simulink model "version5"  (R2018b)
settings: Solver=FixedStepAuto  StartTime=0.0  StopTime=1  FixedStep=0.0005  RelTol=1e-3  EnableMultiTasking=on
model workspace (MAT data in the model file):
  APPS_1_X = [526 863 1200 1537 1837 2212 2310]
  APPS_2_X = [0 342 684 1026 1368 1710 1805]
  APPS_Y = [100 80 60 40 20 0 0]
  Motor_Temp = [0 25 50 75 85 100 115 125 150 175 200 225 250]
  duty_time = [0 1000 5000 6500 7500 9000 10000 10000 10000 10000 10000 10000 10000]
undefined symbols (not defined in the file): I_AN06_5V, I_AN08_5V, I_AN09_5V, I_HALL1, I_SW11_H, O_PWM1_LS0A7, O_PWM2_LS0A7, O_SW01_LS0A4
libraries: ec5744lib x55, simulink x28, canmsglib x12, fuzblock x2
(part 1 of 3)
settings Model: Creator=Hiro  LastModifiedBy=Hiro
settings SolverCC: AutoInsertRateTranBlk=on
settings DataIOCC: LimitDataPoints=on  SaveFormat=Array
settings OptimizationCC: DefaultParameterBehavior=Inlined  InlineInvariantSignals=on  EnhancedBackFolding=on  ExpressionFolding=off  PassReuseOutputArgsAs=Individual arguments  RollThreshold=65  StateBitsets=on  DataBitsets=on  ZeroExternalMemoryAtStartup=off  ZeroInternalMemoryAtStartup=off  EfficientFloat2IntCast=on  OptimizeBlockOrder=speed  DifferentSizesBufferReuse=on
settings DebuggingCC: SolverPrmCheckMsg=warning  InheritedTsInSrcMsg=none  ParameterTunabilityLossMsg=error  SFUnexpectedBacktrackingDiag=warning  SFNoUnconditionalDefaultTransitionDiag=warning  SFExecutionAtInitializationDiag=none
settings HardwareCC: ProdBitPerPointer=32  ProdBitPerSizeT=32  ProdBitPerPtrDiffT=32  ProdLargestAtomicInteger=Long  ProdLargestAtomicFloat=Double  ProdEndianess=BigEndian  ProdWordSize=32  ProdHWDeviceType=Freescale MPC5500
settings ModelReferenceCC: PropagateSignalLabelsOutOfModel=off
settings SFSimCC: SimUseLocalCustomCode=off  MATLABDynamicMemAlloc=off
settings RTWCC: SystemTargetFile=ec5744.tlc  MakeCommand=make_rtw optimized_fixed_point=1  GenerateMakefile=off  TemplateMakefile=ec5744_lcc.tmf  Description=Target for EC5744  GenerateReport=on  RTWUseLocalCustomCode=off  IncludeHyperlinkInReport=on  LaunchReport=on  GenerateTraceInfo=on  GenerateTraceReport=on  GenerateTraceReportSl=on  GenerateTraceReportSf=on  GenerateTraceReportEml=on
settings CodeAppCC: ForceParamTrailComments=on  IgnoreCustomStorageClasses=off  OperatorAnnotations=on  SimulinkDataObjDesc=on  SFDataObjDesc=on  InsertBlockDesc=on
settings STFCustomTargetCC: MultiwordLength=256  ModelReferenceCompliant=off  IncludeMdlTerminateFcn=off  CombineOutputUpdateFcns=on  SuppressErrorStatus=on  ERTCustomFileBanners=on  SupportContinuousTime=off  SupportNonInlinedSFcns=off  RemoveResetFunc=on  MATLABClassNameForMDSCustomization=Simulink.SoftwareTarget.ERTCustomization  SystemTargetFile=ec5744.tlc
settings ERTTargetCC: ModelReferenceCompliant=off  ParMdlRefBuildCompliant=off  CompOptLevelCompliant=off  ConcurrentExecutionCompliant=off  IncludeMdlTerminateFcn=off  SuppressErrorStatus=on  ModelStepFunctionPrototypeControlCompliant=off  CPPClassGenCompliant=off  UseToolchainInfoCompliant=off  GenerateASAP2=on  InlinedParameterPlacement=NonHierarchical  ERTSrcFileBannerTemplate=ec5744_code_template.cgt  ERTHdrFileBannerTemplate=ec5744_code_template.cgt  ERTDataSrcFileTemplate=ec5744_code_template.cgt  ERTDataHdrFileTemplate=ec5744_code_template.cgt  ERTCustomFileTemplate=ec5744_file_process.tlc
settings ConfigComp: CovMetricSettings=dw  CovHtmlReporting=on  CovSaveCumulativeToWorkspaceVar=on  CovSaveSingleToWorkspaceVar=on  CovExternalEMLEnable=off  CovSFcnEnable=off

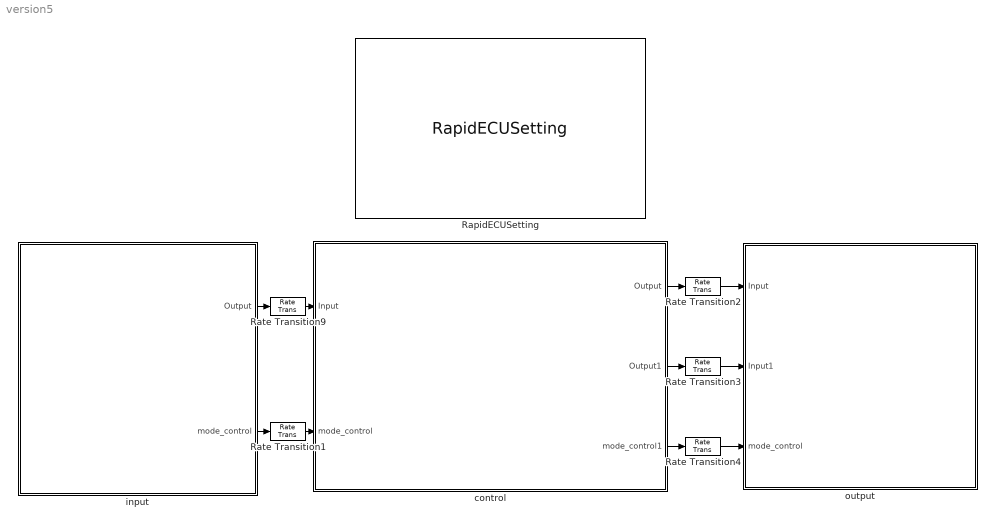
== system version5 ==
  RapidECUSetting : ec5744lib/RapidECU_U3/RapidECUSetting
      settings: SourceProductName=ECUCoder for MPC5744
  Rate Transition{1..4,9} (5 alike) : RateTransition  Integrity=off
  control : Subsystem
  input : Subsystem
  output : Subsystem
  wires:
  control/1(Output) -> Rate Transition2/1
  control/3(mode_control1) -> Rate Transition4/1
  control/2(Output1) -> Rate Transition3/1
  input/1(Output) -> Rate Transition9/1
  Rate Transition9/1 -> control/1(Input)
  input/2(mode_control) -> Rate Transition1/1
  Rate Transition1/1 -> control/2(mode_control)
  Rate Transition2/1 -> output/1(Input)
  Rate Transition3/1 -> output/2(Input1)
  Rate Transition4/1 -> output/3(mode_control)

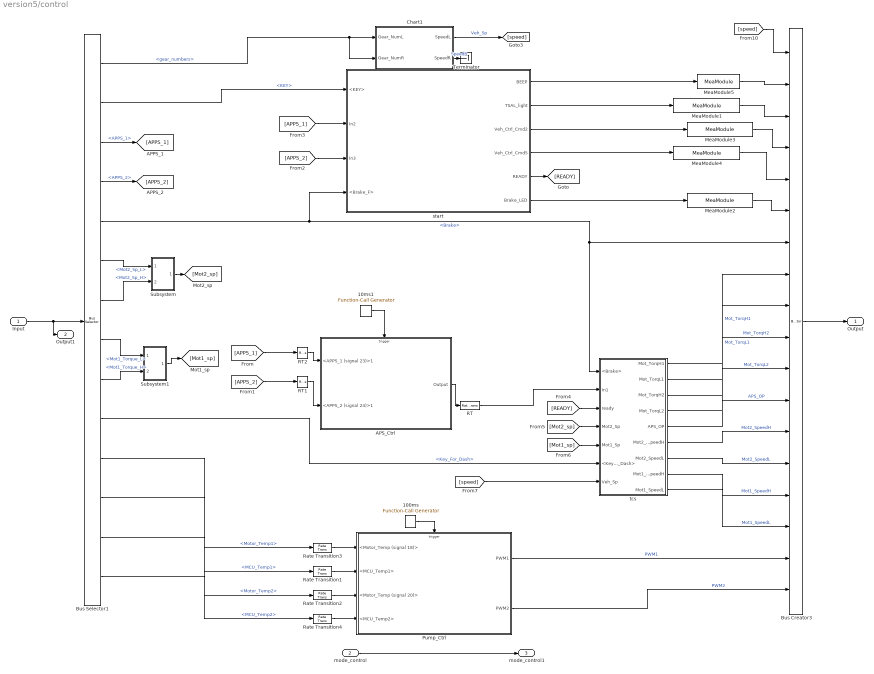
== system version5/control ==
  Input : Inport
  mode_control : Inport  Port=2
  100ms : simulink/Ports & Subsystems/Function-Call Generator  sample_time=0.1  numberOfIterations=1
  10ms1 : simulink/Ports & Subsystems/Function-Call Generator  sample_time=0.01  numberOfIterations=1
  APS_Ctrl : Subsystem
  Bus Creator3 : BusCreator  Inputs=18
  Bus Selector1 : BusSelector  OutputSignals=gear_numbers,KEY,APPS_1,APPS_2,Brake,Mot2_Sp_L,Mot2_Sp_H,Mot1_Torque_L,Mot1_Torque_H,Key_For_Dash,Motor_Temp1,MCU_Temp1,Motor_Temp2,MCU_Temp2
  Chart1 : Stateflow chart  TreatAsAtomicUnit=on
  MeaModule1 : ec5744lib/RapidECU_U3/07Calibration/MeaModule  signal=TSAL_LIGHT
      settings: SourceProductName=ECUCoder for MPC5744
  MeaModule2 : ec5744lib/RapidECU_U3/07Calibration/MeaModule  signal=Brake_LED
      settings: SourceProductName=ECUCoder for MPC5744
  MeaModule3 : ec5744lib/RapidECU_U3/07Calibration/MeaModule  signal=Veh_Ctrl_Cmd2
      settings: SourceProductName=ECUCoder for MPC5744
  MeaModule4 : ec5744lib/RapidECU_U3/07Calibration/MeaModule  signal=Veh_Ctrl_Cmd5
      settings: SourceProductName=ECUCoder for MPC5744
  MeaModule5 : ec5744lib/RapidECU_U3/07Calibration/MeaModule  signal=BEEP
      settings: SourceProductName=ECUCoder for MPC5744
  Pump_Ctrl : Subsystem
  RT : RateTransition  OutPortSampleTime=0.0005
  RT1 : RateTransition  OutPortSampleTime=0.01
  RT2 : RateTransition  OutPortSampleTime=0.01
  Rate Transition{1..4} (4 alike) : RateTransition  Integrity=off
  Subsystem : Subsystem
  Subsystem1 : Subsystem
  Terminator : Terminator
  start : Subsystem
  tcs : Subsystem
  Output : Outport
  Output1 : Outport  Port=2
  mode_control1 : Outport  Port=3
  wires:
  Pump_Ctrl/1(PWM1) -> Bus Creator3/17  "PWM1"
  Pump_Ctrl/2(PWM2) -> Bus Creator3/18  "PWM2"
  Input/1 -> Bus Selector1/1, Output1/1
  MeaModule1/1 -> Bus Creator3/3
  MeaModule2/1 -> Bus Creator3/6
  [APPS_1] -> RT2/1
  [APPS_2] -> RT1/1
  Bus Creator3/1 -> Output/1
  Bus Selector1/5 -> tcs/1(<Brake>), Bus Creator3/7, start/4(<Brake_F>)  "<Brake>"
  Bus Selector1/3 -> [APPS_1]  "<APPS_1>"
  Bus Selector1/4 -> [APPS_2]  "<APPS_2>"
  Bus Selector1/11 -> Rate Transition3/1  "<Motor_Temp1>"
  Bus Selector1/13 -> Rate Transition2/1  "<Motor_Temp2>"
  MeaModule3/1 -> Bus Creator3/4
  MeaModule4/1 -> Bus Creator3/5
  10ms1/1 -> APS_Ctrl/Trigger
  Bus Selector1/12 -> Rate Transition1/1  "<MCU_Temp1>"
  Bus Selector1/14 -> Rate Transition4/1  "<MCU_Temp2>"
  MeaModule5/1 -> Bus Creator3/2
  Bus Selector1/10 -> tcs/6(<Key_For_Dash>)  "<Key_For_Dash>"
  Bus Selector1/6 -> Subsystem/1(<Mot2_Sp_L>)  "<Mot2_Sp_L>"
  Bus Selector1/7 -> Subsystem/2(<Mot2_Sp_H>)  "<Mot2_Sp_H>"
  Bus Selector1/8 -> Subsystem1/1(<Mot1_Sp_L>)  "<Mot1_Torque_L>"
  Bus Selector1/9 -> Subsystem1/2(<Mot1_Sp_H>)  "<Mot1_Torque_H>"
  RT/1 -> tcs/2(In1)
  [READY] -> tcs/3(ready)
  [speed] -> tcs/7(Veh_Sp)
  tcs/1(Mot_TorqH1) -> Bus Creator3/8  "Mot_TorqH1"
  tcs/2(Mot_TorqL1) -> Bus Creator3/9  "Mot_TorqL1"
  tcs/5(APS_OP) -> Bus Creator3/12  "APS_OP"
  Subsystem/1(Mot2_Sp) -> [Mot2_sp]
  Subsystem1/1(Mot1_Sp) -> [Mot1_sp]
  [Mot2_sp] -> tcs/4(Mot2_Sp)
  [Mot1_sp] -> tcs/5(Mot1_Sp)
  mode_control/1 -> mode_control1/1
  tcs/6(Mot2_SpeedH) -> Bus Creator3/13  "Mot2_SpeedH"
  tcs/7(Mot2_SpeedL) -> Bus Creator3/14  "Mot2_SpeedL"
  tcs/8(Mot1_SpeedH) -> Bus Creator3/15  "Mot1_SpeedH"
  tcs/9(Mot1_SpeedL) -> Bus Creator3/16  "Mot1_SpeedL"
  100ms/1 -> Pump_Ctrl/Trigger
  Rate Transition3/1 -> Pump_Ctrl/1(<Motor_Temp (signal 18)>)
  Rate Transition1/1 -> Pump_Ctrl/2(<MCU_Temp1>)
  Rate Transition2/1 -> Pump_Ctrl/3(<Motor_Temp (signal 20)>)
  Rate Transition4/1 -> Pump_Ctrl/4(<MCU_Temp2>)
  Bus Selector1/2 -> start/1(<KEY>)  "<KEY>"
  [APPS_1] -> start/2(In2)
  [APPS_2] -> start/3(In3)
  start/1(BEEP) -> MeaModule5/1
  start/2(TSAL_light) -> MeaModule1/1
  start/3(Veh_Ctrl_Cmd2) -> MeaModule3/1
  start/4(Veh_Ctrl_Cmd5) -> MeaModule4/1
  start/5(READY) -> [READY]
  Chart1/1(SpeedL) -> [speed]  "Veh_Sp"
  [speed] -> Bus Creator3/1
  start/6(Brake_LED) -> MeaModule2/1
  tcs/3(Mot_TorqH2) -> Bus Creator3/10  "Mot_TorqH2"
  tcs/4(Mot_TorqL2) -> Bus Creator3/11  "Mot_TorqL2"
  APS_Ctrl/1(Output) -> RT/1
  RT1/1 -> APS_Ctrl/2(<APPS_2 (signal 24)>1)
  RT2/1 -> APS_Ctrl/1(<APPS_1 (signal 23)>1)
  Bus Selector1/1 -> Chart1/2(Gear_NumR), Chart1/1(Gear_NumL)  "<gear_numbers>"
  Chart1/2(SpeedR) -> Terminator/1  "SpeedR"

== system version5/input ==
  note: AnalogInput
  note: DASHtoVCU
  note: MCUtoVCU2
  note: BMStoVCU
  note: MCU to VCU1
  AnalogInput : Subsystem
  BMStoVCU : Subsystem
  Bus Creator : BusCreator  Inputs=27
  DASHtoVCU : Subsystem
  FrequencyRead1 : ec5744lib/RapidECU_U3/01BasicInput/FrequencyRead  channel=37:I_HALL1  sampletime=-1
      settings: SourceProductName=ECUCoder for MPC5744
  MCU to VCU : Subsystem
  MCUtoVCU : Subsystem
  SwitchInput : ec5744lib/RapidECU_U3/01BasicInput/SwitchInput  channel=44:I_SW11_H  sampletime=-1
      settings: SourceProductName=ECUCoder for MPC5744
  Output : Outport
  mode_control : Outport  Port=2
  wires:
  SwitchInput/1 -> Bus Creator/26  "KEY"
  Bus Creator/1 -> Output/1
  AnalogInput/1(Brake) -> Bus Creator/23
  AnalogInput/2(APPS_1) -> Bus Creator/24
  AnalogInput/3(APPS_2) -> Bus Creator/25
  MCU to VCU/1(Mot2_Sp_H) -> Bus Creator/1
  MCU to VCU/2(Mot2_Sp_L) -> Bus Creator/2
  MCU to VCU/3(Mot2_Torque_H) -> Bus Creator/3
  MCU to VCU/4(Mot2_Torque_L) -> Bus Creator/4
  MCU to VCU/5(Mot1_Sp_H) -> Bus Creator/5
  MCU to VCU/6(Mot1_Sp_L) -> Bus Creator/6
  MCU to VCU/7(Mot1_Torque_H) -> Bus Creator/7
  MCU to VCU/8(Mot1_Torque_L) -> Bus Creator/8
  MCU to VCU/9(mode_control) -> mode_control/1
  MCUtoVCU/1(MCU_Temp1) -> Bus Creator/17
  MCUtoVCU/2(Motor_Temp1) -> Bus Creator/18
  MCUtoVCU/3(MCU_Temp2) -> Bus Creator/19
  MCUtoVCU/4(Motor_Temp2) -> Bus Creator/20
  BMStoVCU/1(Bat_Max_Temp) -> Bus Creator/9
  BMStoVCU/2(Bat_Ala_Lv) -> Bus Creator/10
  BMStoVCU/3(Bat_Current_LSB) -> Bus Creator/11
  BMStoVCU/4(Bat_Current_MSB) -> Bus Creator/12
  BMStoVCU/5(Bat_Stat) -> Bus Creator/13
  BMStoVCU/6(Bat_Voltage_LSB) -> Bus Creator/14
  BMStoVCU/7(Bat_Valtage_MSB) -> Bus Creator/15
  BMStoVCU/8(Bat_soc) -> Bus Creator/16
  DASHtoVCU/1(GEAR) -> Bus Creator/21
  DASHtoVCU/2(Key_For_Dash) -> Bus Creator/22
  FrequencyRead1/1 -> Bus Creator/27  "gear_numbers"

== system version5/output ==
  note: PWMOutput
  note: SwitchOutput
  note: VCUtoDASH
  note: VCUtoMCU
  Input : Inport
  Input1 : Inport  Port=2
  mode_control : Inport  Port=3
  Bus Selector : BusSelector  OutputSignals=BEEP,TSAL_LIGHT,Brake_LED
  Bus Selector6 : BusSelector  OutputSignals=PWM1,PWM2
  Constant16 : Constant  Value=100  OutDataTypeStr=uint16
  Constant17 : Constant  Value=100  OutDataTypeStr=uint16
  PowerDriverPWM : ec5744lib/RapidECU_U3/03PowerDriverPWM/PowerDriverPWM  channel=60:O_PWM1_LS0A7  sampletime=-1
      settings: SourceProductName=ECUCoder for MPC5744
  PowerDriverPWM1 : ec5744lib/RapidECU_U3/03PowerDriverPWM/PowerDriverPWM  channel=90:O_PWM2_LS0A7  sampletime=-1
      settings: SourceProductName=ECUCoder for MPC5744
  PowerDriverSwitch(LS) : ec5744lib/RapidECU_U3/02PowerDriverSwitch/PowerDriverSwitch(LS)  channel=58:O_SW01_LS0A4  sampletime=-1
      settings: SourceProductName=ECUCoder for MPC5744
  PowerDriverSwitch(LS)1 : ec5744lib/RapidECU_U3/02PowerDriverSwitch/PowerDriverSwitch(LS)  channel=58:O_SW01_LS0A4  sampletime=-1
      settings: SourceProductName=ECUCoder for MPC5744
  PowerDriverSwitch(LS)2 : ec5744lib/RapidECU_U3/02PowerDriverSwitch/PowerDriverSwitch(LS)  channel=58:O_SW01_LS0A4  sampletime=-1
      settings: SourceProductName=ECUCoder for MPC5744
  Subsystem : Subsystem
  VCUtoMCU : Subsystem
  wires:
  Bus Selector6/1 -> PowerDriverPWM/2  "<PWM1>"
  Bus Selector6/2 -> PowerDriverPWM1/2  "<PWM2>"
  Input/1 -> Subsystem/1(In1), VCUtoMCU/1(In1), Bus Selector6/1, Bus Selector/1
  Bus Selector/1 -> PowerDriverSwitch(LS)2/1  "<BEEP>"
  Bus Selector/3 -> PowerDriverSwitch(LS)/1  "<Brake_LED>"
  Constant17/1 -> PowerDriverPWM/1
  Constant16/1 -> PowerDriverPWM1/1
  Bus Selector/2 -> PowerDriverSwitch(LS)1/1  "<TSAL_LIGHT>"
  mode_control/1 -> Subsystem/2(mode_control)
  Input1/1 -> Subsystem/3(In4)

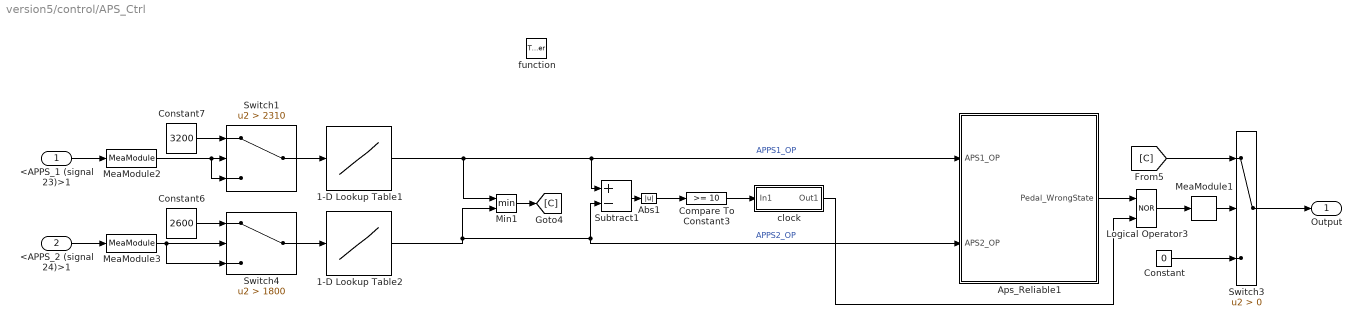
== system version5/control/APS_Ctrl ==
  <APPS_1 (signal 23)>1 : Inport
  <APPS_2 (signal 24)>1 : Inport  Port=2
  function : TriggerPort  TriggerType=function-call  VariantControl=Variant
  1-D Lookup Table1 : Lookup_n-D  NumberOfTableDimensions=1  BreakpointsForDimension1=APPS_1_X  Table=APPS_Y  ExtrapMethod=Clip  InternalRulePriority=Speed  OutDataTypeStr=uint8  RndMeth=Simplest  InputSameDT=on
  1-D Lookup Table2 : Lookup_n-D  NumberOfTableDimensions=1  BreakpointsForDimension1=APPS_2_X  Table=APPS_Y  ExtrapMethod=Clip  InternalRulePriority=Speed  OutDataTypeStr=uint8  RndMeth=Simplest  InputSameDT=on
  Abs1 : Abs  OutDataTypeStr=uint16
      settings: LockScale=on
  Aps_Reliable1 : Stateflow chart  TreatAsAtomicUnit=on
  Compare To Constant3 : simulink/Logic and Bit Operations/Compare To Constant  relop=>=  const=10  OutDataTypeStr=boolean
  Constant : Constant  Value=0
  Constant6 : Constant  Value=2600  OutDataTypeStr=uint16
  Constant7 : Constant  Value=3200  OutDataTypeStr=uint16
  Logical Operator3 : Logic  Operator=NOR  AllPortsSameDT=off  OutDataTypeStr=boolean
  MeaModule1 : ec5744lib/RapidECU_U3/07Calibration/MeaModule  signal=Mot_Torq
      settings: SourceProductName=ECUCoder for MPC5744
  MeaModule2 : ec5744lib/RapidECU_U3/07Calibration/MeaModule  signal=APS1
      settings: SourceProductName=ECUCoder for MPC5744
  MeaModule3 : ec5744lib/RapidECU_U3/07Calibration/MeaModule  signal=APS2
      settings: SourceProductName=ECUCoder for MPC5744
  Min1 : MinMax  Inputs=2
  Subtract1 : Sum  Inputs=+-  AccumDataTypeStr=double  OutDataTypeStr=uint16  SaturateOnIntegerOverflow=on
  Switch1 : Switch  Criteria=u2 > Threshold  Threshold=2310
  Switch3 : Switch  Criteria=u2 > Threshold  OutDataTypeStr=uint16
  Switch4 : Switch  Criteria=u2 > Threshold  Threshold=1800
  clock : Subsystem
  Output : Outport
  wires:
  Subtract1/1 -> Abs1/1
  Min1/1 -> [C]
  <APPS_1 (signal 23)>1/1 -> MeaModule2/1
  <APPS_2 (signal 24)>1/1 -> MeaModule3/1
  [C] -> Switch3/1
  Constant6/1 -> Switch4/1
  Constant7/1 -> Switch1/1
  MeaModule2/1 -> Switch1/3, Switch1/2
  MeaModule3/1 -> Switch4/3, Switch4/2
  Logical Operator3/1 -> MeaModule1/1
  Constant/1 -> Switch3/3
  MeaModule1/1 -> Switch3/2
  Aps_Reliable1/1(Pedal_WrongState) -> Logical Operator3/1
  Switch1/1 -> 1-D Lookup Table1/1
  Switch4/1 -> 1-D Lookup Table2/1
  1-D Lookup Table1/1 -> Min1/1, Subtract1/1, Aps_Reliable1/1(APS1_OP)  "APPS1_OP"
  1-D Lookup Table2/1 -> Min1/2, Subtract1/2, Aps_Reliable1/2(APS2_OP)  "APPS2_OP"
  Switch3/1 -> Output/1
  Compare To Constant3/1 -> clock/1(In1)
  Abs1/1 -> Compare To Constant3/1
  clock/1(Out1) -> Logical Operator3/2

== system version5/control/Pump_Ctrl ==
  <Motor_Temp (signal 18)> : Inport
  <MCU_Temp1> : Inport  Port=2
  <Motor_Temp (signal 20)> : Inport  Port=3
  <MCU_Temp2> : Inport  Port=4
  function : TriggerPort  TriggerType=function-call  VariantControl=Variant
  1-D Lookup Table : Lookup_n-D  NumberOfTableDimensions=1  BreakpointsForDimension1=Motor_Temp  Table=duty_time  InternalRulePriority=Speed  RndMeth=Simplest  InputSameDT=on
  1-D Lookup Table1 : Lookup_n-D  NumberOfTableDimensions=1  BreakpointsForDimension1=Motor_Temp  Table=duty_time  InternalRulePriority=Speed  RndMeth=Simplest  InputSameDT=on
  Data Type Conversion : DataTypeConversion  OutDataTypeStr=uint16
  Data Type Conversion1 : DataTypeConversion  OutDataTypeStr=uint16
  Max : MinMax  Function=max  Inputs=2  OutDataTypeStr=double
  Max1 : MinMax  Function=max  Inputs=2  OutDataTypeStr=double
  MeaModule : ec5744lib/RapidECU_U3/07Calibration/MeaModule  signal=duty_time18
      settings: SourceProductName=ECUCoder for MPC5744
  MeaModule1 : ec5744lib/RapidECU_U3/07Calibration/MeaModule  signal=duty_time20
      settings: SourceProductName=ECUCoder for MPC5744
  PWM1 : Outport
  PWM2 : Outport  Port=2
  wires:
  Data Type Conversion/1 -> MeaModule/1
  1-D Lookup Table/1 -> Data Type Conversion/1  "duty_time_18"
  1-D Lookup Table1/1 -> Data Type Conversion1/1  "duty_time_20"
  Data Type Conversion1/1 -> MeaModule1/1
  MeaModule/1 -> PWM1/1
  MeaModule1/1 -> PWM2/1
  Max1/1 -> 1-D Lookup Table1/1
  Max/1 -> 1-D Lookup Table/1
  <Motor_Temp (signal 20)>/1 -> Max1/1
  <MCU_Temp2>/1 -> Max1/2
  <Motor_Temp (signal 18)>/1 -> Max/1
  <MCU_Temp1>/1 -> Max/2

== system version5/control/Subsystem ==
  <Mot2_Sp_L> : Inport
  <Mot2_Sp_H> : Inport  Port=2
  Add : Sum
  Data Type Conversion4 : DataTypeConversion  OutDataTypeStr=uint16
  Data Type Conversion5 : DataTypeConversion  OutDataTypeStr=uint16
  Shift Arithmetic : ArithShift  BitShiftNumber=8  BitShiftDirection=Left
  Mot2_Sp : Outport
  wires:
  <Mot2_Sp_H>/1 -> Data Type Conversion4/1
  Data Type Conversion5/1 -> Add/1
  Data Type Conversion4/1 -> Shift Arithmetic/1
  Shift Arithmetic/1 -> Add/2
  Add/1 -> Mot2_Sp/1
  <Mot2_Sp_L>/1 -> Data Type Conversion5/1

== system version5/control/Subsystem1 ==
  <Mot1_Sp_L> : Inport
  <Mot1_Sp_H> : Inport  Port=2
  Add : Sum
  Data Type Conversion4 : DataTypeConversion  OutDataTypeStr=uint16
  Data Type Conversion5 : DataTypeConversion  OutDataTypeStr=uint16
  Shift Arithmetic : ArithShift  BitShiftNumber=8  BitShiftDirection=Left
  Mot1_Sp : Outport
  wires:
  <Mot1_Sp_L>/1 -> Data Type Conversion5/1
  Add/1 -> Mot1_Sp/1
  Shift Arithmetic/1 -> Add/2
  Data Type Conversion4/1 -> Shift Arithmetic/1
  Data Type Conversion5/1 -> Add/1
  <Mot1_Sp_H>/1 -> Data Type Conversion4/1

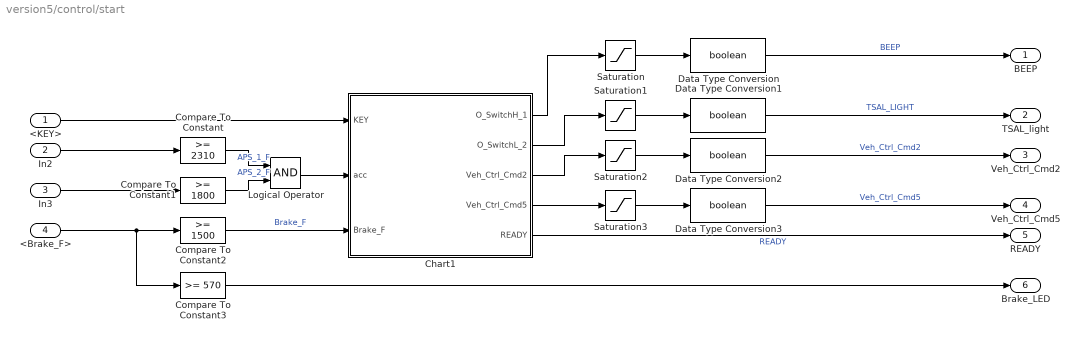
== system version5/control/start ==
  <KEY> : Inport
  In2 : Inport  Port=2
  In3 : Inport  Port=3
  <Brake_F> : Inport  Port=4
  Chart1 : Stateflow chart  TreatAsAtomicUnit=on
  Compare To Constant : simulink/Logic and Bit Operations/Compare To Constant  relop=>=  const=2310  OutDataTypeStr=boolean
  Compare To Constant1 : simulink/Logic and Bit Operations/Compare To Constant  relop=>=  const=1800  OutDataTypeStr=boolean
  Compare To Constant2 : simulink/Logic and Bit Operations/Compare To Constant  relop=>=  const=1500  OutDataTypeStr=boolean
  Compare To Constant3 : simulink/Logic and Bit Operations/Compare To Constant  relop=>=  const=570  OutDataTypeStr=boolean
  Data Type Conversion{,1..3} (4 alike) : DataTypeConversion  OutDataTypeStr=boolean
  Logical Operator : Logic  AllPortsSameDT=off  OutDataTypeStr=boolean
  Saturation{,1..3} (4 alike) : Saturate  UpperLimit=1  LowerLimit=0  OutDataTypeStr=uint8
  BEEP : Outport
  TSAL_light : Outport  Port=2
  Veh_Ctrl_Cmd2 : Outport  Port=3
  Veh_Ctrl_Cmd5 : Outport  Port=4
  READY : Outport  Port=5
  Brake_LED : Outport  Port=6
  wires:
  Chart1/1(O_SwitchH_1) -> Saturation/1
  Compare To Constant1/1 -> Logical Operator/2  "APS_2_F"
  Chart1/3(Veh_Ctrl_Cmd2) -> Saturation2/1
  Chart1/2(O_SwitchL_2) -> Saturation1/1
  Saturation/1 -> Data Type Conversion/1
  Saturation1/1 -> Data Type Conversion1/1
  Compare To Constant/1 -> Logical Operator/1  "APS_1_F"
  In2/1 -> Compare To Constant/1
  Chart1/4(Veh_Ctrl_Cmd5) -> Saturation3/1
  Saturation3/1 -> Data Type Conversion3/1
  Saturation2/1 -> Data Type Conversion2/1
  Logical Operator/1 -> Chart1/2(acc)
  Chart1/5(READY) -> READY/1  "READY"
  In3/1 -> Compare To Constant1/1
  <Brake_F>/1 -> Compare To Constant3/1, Compare To Constant2/1
  Data Type Conversion3/1 -> Veh_Ctrl_Cmd5/1  "Veh_Ctrl_Cmd5"
  Data Type Conversion1/1 -> TSAL_light/1  "TSAL_LIGHT"
  Data Type Conversion2/1 -> Veh_Ctrl_Cmd2/1  "Veh_Ctrl_Cmd2"
  Data Type Conversion/1 -> BEEP/1  "BEEP"
  <KEY>/1 -> Chart1/1(KEY)
  Compare To Constant2/1 -> Chart1/3(Brake_F)  "Brake_F"
  Compare To Constant3/1 -> Brake_LED/1

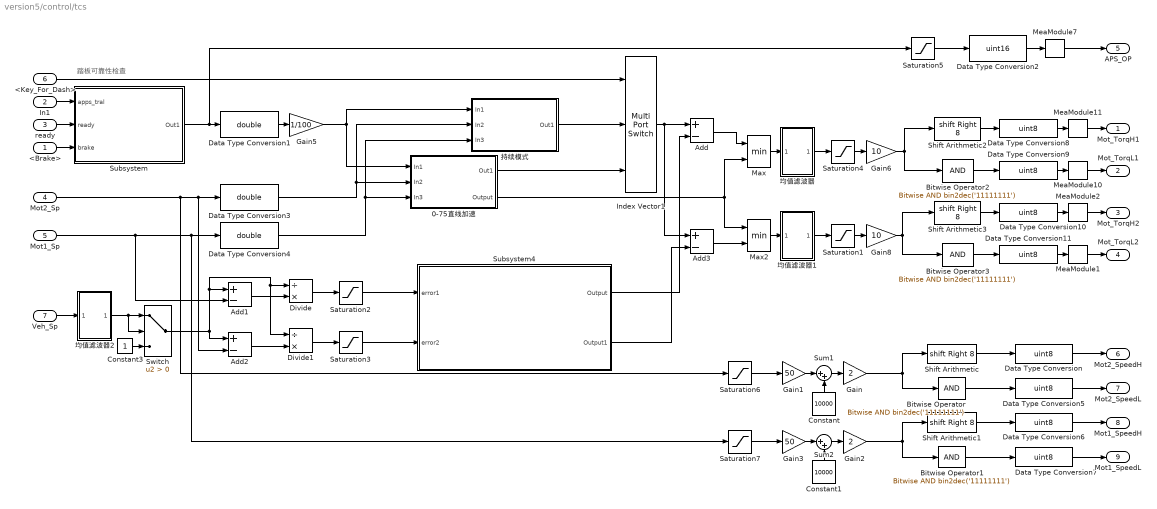
== system version5/control/tcs ==
  note: 踏板可靠性检查
  <Brake> : Inport
  In1 : Inport  Port=2
  ready : Inport  Port=3
  Mot2_Sp : Inport  Port=4
  Mot1_Sp : Inport  Port=5
  <Key_For_Dash> : Inport  Port=6
  Veh_Sp : Inport  Port=7
  0-75直线加速 : Subsystem
  Add : Sum  Inputs=+-  AccumDataTypeStr=double  OutDataTypeStr=double
  Add1 : Sum  Inputs=+-
  Add2 : Sum  Inputs=+-
  Add3 : Sum  Inputs=+-  AccumDataTypeStr=double  OutDataTypeStr=double
  Bitwise Operator{,1..3} (4 alike) : simulink/Logic and Bit Operations/Bitwise Operator  logicop=AND  UseBitMask=on  BitMask=bin2dec('11111111')  BitMaskRealWorld=Stored Integer
  Constant : Constant  Value=10000  OutDataTypeStr=uint16
  Constant1 : Constant  Value=10000  OutDataTypeStr=uint16
  Constant3 : Constant
  Data Type Conversion{,5..11} (8 alike) : DataTypeConversion  OutDataTypeStr=uint8
  Data Type Conversion1 : DataTypeConversion  OutDataTypeStr=double
  Data Type Conversion2 : DataTypeConversion  OutDataTypeStr=uint16
  Data Type Conversion3 : DataTypeConversion  OutDataTypeStr=double
  Data Type Conversion4 : DataTypeConversion  OutDataTypeStr=double  LockScale=on
  Divide : Product  Inputs=/*
  Divide1 : Product  Inputs=/*
  Gain : Gain  Gain=2  OutDataTypeStr=uint16
  Gain1 : Gain  Gain=50  OutDataTypeStr=uint16
  Gain2 : Gain  Gain=2  OutDataTypeStr=uint16
  Gain3 : Gain  Gain=50  OutDataTypeStr=uint16
  Gain5 : Gain  Gain=1/100  OutDataTypeStr=double
  Gain6 : Gain  Gain=10  OutDataTypeStr=uint16
  Gain8 : Gain  Gain=10  OutDataTypeStr=uint16
  Index Vector1 : MultiPortSwitch  DataPortOrder=Zero-based contiguous  Inputs=2  zeroidx=on  OutDataTypeStr=double
  Max : MinMax  Inputs=2
  Max2 : MinMax  Inputs=2
  MeaModule1 : ec5744lib/RapidECU_U3/07Calibration/MeaModule  signal=Mot_TorqL2
      settings: SourceProductName=ECUCoder for MPC5744
  MeaModule10 : ec5744lib/RapidECU_U3/07Calibration/MeaModule  signal=Mot_TorqL1
      settings: SourceProductName=ECUCoder for MPC5744
  MeaModule11 : ec5744lib/RapidECU_U3/07Calibration/MeaModule  signal=Mot_TorqH1
      settings: SourceProductName=ECUCoder for MPC5744
  MeaModule2 : ec5744lib/RapidECU_U3/07Calibration/MeaModule  signal=Mot_TorqH2
      settings: SourceProductName=ECUCoder for MPC5744
  MeaModule7 : ec5744lib/RapidECU_U3/07Calibration/MeaModule  signal=APS_OP
      settings: SourceProductName=ECUCoder for MPC5744
  Saturation1 : Saturate  UpperLimit=140  LowerLimit=0
  Saturation2 : Saturate  UpperLimit=0.8  LowerLimit=0
  Saturation3 : Saturate  UpperLimit=0.8  LowerLimit=0
  Saturation4 : Saturate  UpperLimit=140  LowerLimit=0
  Saturation5 : Saturate  UpperLimit=100  LowerLimit=0
  Saturation6 : Saturate  UpperLimit=100  LowerLimit=0
  Saturation7 : Saturate  UpperLimit=100  LowerLimit=0
  Shift Arithmetic{,1..3} (4 alike) : ArithShift  BitShiftNumber=8  BitShiftDirection=Right
  Subsystem : Subsystem
  Subsystem4 : Subsystem
  Sum1 : Sum  Inputs=|++
  Sum2 : Sum  Inputs=|++
  Switch : Switch  Criteria=u2 > Threshold
  均值滤波器 : Subsystem
  均值滤波器1 : Subsystem
  均值滤波器2 : Subsystem
  持续模式 : Subsystem
  Mot_TorqH1 : Outport  OutDataTypeStr=uint8
  Mot_TorqL1 : Outport  Port=2  OutDataTypeStr=uint8
  Mot_TorqH2 : Outport  Port=3  OutDataTypeStr=uint8
  Mot_TorqL2 : Outport  Port=4  OutDataTypeStr=uint8
  APS_OP : Outport  Port=5  OutDataTypeStr=uint16
  Mot2_SpeedH : Outport  Port=6  OutDataTypeStr=uint8
  Mot2_SpeedL : Outport  Port=7  OutDataTypeStr=uint8
  Mot1_SpeedH : Outport  Port=8  OutDataTypeStr=uint8
  Mot1_SpeedL : Outport  Port=9  OutDataTypeStr=uint8
  wires:
  Data Type Conversion8/1 -> MeaModule11/1
  MeaModule10/1 -> Mot_TorqL1/1
  Data Type Conversion9/1 -> MeaModule10/1
  MeaModule11/1 -> Mot_TorqH1/1
  In1/1 -> Subsystem/1(apps_tral)
  ready/1 -> Subsystem/2(ready)
  <Brake>/1 -> Subsystem/3(brake)
  <Key_For_Dash>/1 -> Index Vector1/1
  Data Type Conversion2/1 -> MeaModule7/1
  MeaModule7/1 -> APS_OP/1
  Data Type Conversion1/1 -> Gain5/1
  Data Type Conversion3/1 -> 持续模式/2(In2), 0-75直线加速/2(In2)
  Data Type Conversion4/1 -> 持续模式/3(In3), 0-75直线加速/3(In3)
  Subsystem/1(Out1) -> Saturation5/1, Data Type Conversion1/1
  Gain5/1 -> 0-75直线加速/1(In1), 持续模式/1(In1)
  持续模式/1(Out1) -> Index Vector1/2
  0-75直线加速/1(Out1) -> Index Vector1/3
  Data Type Conversion5/1 -> Mot2_SpeedL/1
  Data Type Conversion/1 -> Mot2_SpeedH/1
  Mot1_Sp/1 -> Add1/2, Saturation7/1, Data Type Conversion4/1
  Data Type Conversion7/1 -> Mot1_SpeedL/1
  Data Type Conversion6/1 -> Mot1_SpeedH/1
  Index Vector1/1 -> Add3/1, Add/1
  0-75直线加速/2(Output) -> Max/2, Max2/1
  Subsystem4/1(Output) -> Add/2
  Gain1/1 -> Sum1/1
  Constant/1 -> Sum1/2
  Sum1/1 -> Gain/1
  Mot2_Sp/1 -> Add2/2, Data Type Conversion3/1, Saturation6/1
  Bitwise Operator/1 -> Data Type Conversion5/1
  Shift Arithmetic/1 -> Data Type Conversion/1
  Sum2/1 -> Gain2/1
  Constant1/1 -> Sum2/2
  Shift Arithmetic1/1 -> Data Type Conversion6/1
  Bitwise Operator1/1 -> Data Type Conversion7/1
  Gain3/1 -> Sum2/1
  Shift Arithmetic2/1 -> Data Type Conversion8/1
  Bitwise Operator2/1 -> Data Type Conversion9/1
  Add2/1 -> Divide1/2
  Add1/1 -> Divide/2
  Divide/1 -> Saturation2/1
  Divide1/1 -> Saturation3/1
  Subsystem4/2(Output1) -> Add3/2
  Add3/1 -> Max2/2
  Add/1 -> Max/1
  Bitwise Operator3/1 -> Data Type Conversion11/1
  Shift Arithmetic3/1 -> Data Type Conversion10/1
  Gain8/1 -> Shift Arithmetic3/1, Bitwise Operator3/1
  MeaModule2/1 -> Mot_TorqH2/1
  Data Type Conversion11/1 -> MeaModule1/1
  MeaModule1/1 -> Mot_TorqL2/1
  Data Type Conversion10/1 -> MeaModule2/1
  均值滤波器1/1(Out1) -> Saturation1/1
  Max/1 -> 均值滤波器/1(In1)
  Max2/1 -> 均值滤波器1/1(In1)
  均值滤波器/1(Out1) -> Saturation4/1
  Gain6/1 -> Bitwise Operator2/1, Shift Arithmetic2/1
  Saturation4/1 -> Gain6/1
  Saturation1/1 -> Gain8/1
  Gain/1 -> Shift Arithmetic/1, Bitwise Operator/1
  Gain2/1 -> Shift Arithmetic1/1, Bitwise Operator1/1
  Saturation5/1 -> Data Type Conversion2/1
  Saturation6/1 -> Gain1/1
  Saturation7/1 -> Gain3/1
  Saturation2/1 -> Subsystem4/1(error1)
  Saturation3/1 -> Subsystem4/2(error2)
  Veh_Sp/1 -> 均值滤波器2/1(In1)
  Switch/1 -> Add2/1, Add1/1, Divide1/1, Divide/1
  均值滤波器2/1(Out1) -> Switch/1, Switch/2
  Constant3/1 -> Switch/3

== system version5/input/AnalogInput ==
  10ms : simulink/Ports & Subsystems/Function-Call Generator  sample_time=0.01  numberOfIterations=1
  10ms1 : simulink/Ports & Subsystems/Function-Call Generator  sample_time=0.01  numberOfIterations=1
  Acc Pedal Gather : Subsystem
  Brake Pedal Gather : Subsystem
  Brake : Outport
  APPS_1 : Outport  Port=2
  APPS_2 : Outport  Port=3
  wires:
  Brake Pedal Gather/1(Brake) -> Brake/1
  Acc Pedal Gather/1(APPS_1) -> APPS_1/1
  Acc Pedal Gather/2(APPS_2) -> APPS_2/1
  10ms/1 -> Brake Pedal Gather/Trigger
  10ms1/1 -> Acc Pedal Gather/Trigger

== system version5/input/BMStoVCU ==
  CANReceive : ec5744lib/RapidECU_U3/04CANCommunication/CANReceive  canmodule=1  canbuffer=4  canmessageid=hex2dec('186240F3')  canmessagetype=Extended(29-bit ID)  datalength=8  sampletime=-1
      settings: SourceProductName=ECUCoder for MPC5744
  CANReceive1 : ec5744lib/RapidECU_U3/04CANCommunication/CANReceive  canmodule=1  canbuffer=5  canmessageid=hex2dec('186040F3')  canmessagetype=Extended(29-bit ID)  datalength=8  sampletime=-1
      settings: SourceProductName=ECUCoder for MPC5744
  Function-Call Subsystem : Subsystem  TreatAsAtomicUnit=on
  Function-Call Subsystem1 : Subsystem  TreatAsAtomicUnit=on
  Terminator : Terminator
  Terminator1 : Terminator
  Bat_Max_Temp : Outport
  Bat_Ala_Lv : Outport  Port=2
  Bat_Current_LSB : Outport  Port=3
  Bat_Current_MSB : Outport  Port=4
  Bat_Stat : Outport  Port=5
  Bat_Voltage_LSB : Outport  Port=6
  Bat_Valtage_MSB : Outport  Port=7
  Bat_soc : Outport  Port=8
  wires:
  CANReceive/2 -> Function-Call Subsystem/1(CAN_OK)
  CANReceive1/3 -> Function-Call Subsystem1/2(ID)
  CANReceive1/2 -> Function-Call Subsystem1/1(CAN_OK)
  CANReceive1/4 -> Function-Call Subsystem1/3(Msg)
  Function-Call Subsystem/1(Bat_Ala_Lv) -> Bat_Ala_Lv/1  "Bat_Ala_Lv"
  CANReceive/4 -> Function-Call Subsystem/3(Msg)
  CANReceive/5 -> Terminator/1
  CANReceive/1 -> Function-Call Subsystem/Trigger
  CANReceive1/5 -> Terminator1/1
  CANReceive1/1 -> Function-Call Subsystem1/Trigger
  Function-Call Subsystem/4(Bat_Stat) -> Bat_Stat/1  "Bat_Stat"
  Function-Call Subsystem/2(Bat_Current_LSB) -> Bat_Current_LSB/1  "Bat_Current_LSB"
  CANReceive/3 -> Function-Call Subsystem/2(ID)
  Function-Call Subsystem/3(Bat_Current_MSB) -> Bat_Current_MSB/1  "Bat_Current_MSB"
  Function-Call Subsystem/7(Bat_soc) -> Bat_soc/1  "Bat_soc"
  Function-Call Subsystem/6(Bat_Valtage_MSB) -> Bat_Valtage_MSB/1  "Bat_Valtage_MSB"
  Function-Call Subsystem/5(Bat_Voltage_LSB) -> Bat_Voltage_LSB/1  "Bat_Voltage_LSB"
  Function-Call Subsystem1/1(Bat_Max_Temp) -> Bat_Max_Temp/1  "Bat_Max_Temp"

== system version5/input/DASHtoVCU ==
  CANReceive6 : ec5744lib/RapidECU_U3/04CANCommunication/CANReceive  canmodule=1  canbuffer=6  canmessageid=hex2dec('186040F3')  canmessagetype=Extended(29-bit ID)  datalength=8  sampletime=-1
      settings: SourceProductName=ECUCoder for MPC5744
  Function-Call Subsystem6 : Subsystem  TreatAsAtomicUnit=on
  Terminator6 : Terminator
  GEAR : Outport
  Key_For_Dash : Outport  Port=2
  wires:
  CANReceive6/4 -> Function-Call Subsystem6/3(Msg)
  Function-Call Subsystem6/2(Key_For_Dash) -> Key_For_Dash/1  "Key_For_Dash"
  Function-Call Subsystem6/1(GEAR) -> GEAR/1  "GEAR"
  CANReceive6/3 -> Function-Call Subsystem6/2(ID)
  CANReceive6/2 -> Function-Call Subsystem6/1(CAN_OK)
  CANReceive6/1 -> Function-Call Subsystem6/Trigger
  CANReceive6/5 -> Terminator6/1

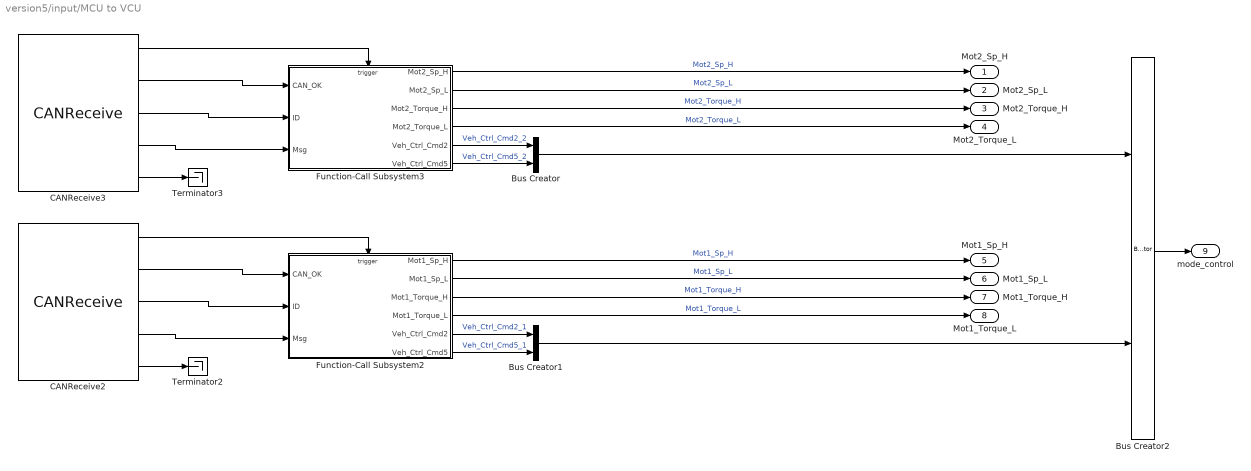
== system version5/input/MCU to VCU ==
  Bus Creator : BusCreator  Inputs=2
  Bus Creator1 : BusCreator  Inputs=2
  Bus Creator2 : BusCreator  Inputs=2
  CANReceive2 : ec5744lib/RapidECU_U3/04CANCommunication/CANReceive  canmodule=0  canbuffer=3  canmessageid=hex2dec('CEFC6EF')  canmessagetype=Extended(29-bit ID)  datalength=8  sampletime=-1
      settings: SourceProductName=ECUCoder for MPC5744
  CANReceive3 : ec5744lib/RapidECU_U3/04CANCommunication/CANReceive  canmodule=0  canbuffer=1  canmessageid=hex2dec('CB221EF')  canmessagetype=Extended(29-bit ID)  datalength=8  sampletime=-1
      settings: SourceProductName=ECUCoder for MPC5744
  Function-Call Subsystem2 : Subsystem  TreatAsAtomicUnit=on
  Function-Call Subsystem3 : Subsystem  TreatAsAtomicUnit=on
  Terminator2 : Terminator
  Terminator3 : Terminator
  Mot2_Sp_H : Outport
  Mot2_Sp_L : Outport  Port=2
  Mot2_Torque_H : Outport  Port=3
  Mot2_Torque_L : Outport  Port=4
  Mot1_Sp_H : Outport  Port=5
  Mot1_Sp_L : Outport  Port=6
  Mot1_Torque_H : Outport  Port=7
  Mot1_Torque_L : Outport  Port=8
  mode_control : Outport  Port=9
  wires:
  CANReceive3/1 -> Function-Call Subsystem3/Trigger
  Function-Call Subsystem3/5(Veh_Ctrl_Cmd2) -> Bus Creator/1  "Veh_Ctrl_Cmd2_2"
  CANReceive2/3 -> Function-Call Subsystem2/2(ID)
  CANReceive2/1 -> Function-Call Subsystem2/Trigger
  CANReceive2/2 -> Function-Call Subsystem2/1(CAN_OK)
  Function-Call Subsystem2/5(Veh_Ctrl_Cmd2) -> Bus Creator1/1  "Veh_Ctrl_Cmd2_1"
  Function-Call Subsystem3/6(Veh_Ctrl_Cmd5) -> Bus Creator/2  "Veh_Ctrl_Cmd5_2"
  CANReceive3/5 -> Terminator3/1
  CANReceive3/3 -> Function-Call Subsystem3/2(ID)
  Function-Call Subsystem2/6(Veh_Ctrl_Cmd5) -> Bus Creator1/2  "Veh_Ctrl_Cmd5_1"
  CANReceive2/5 -> Terminator2/1
  CANReceive2/4 -> Function-Call Subsystem2/3(Msg)
  Function-Call Subsystem2/3(Mot1_Torque_H) -> Mot1_Torque_H/1  "Mot1_Torque_H"
  Function-Call Subsystem3/4(Mot2_Torque_L) -> Mot2_Torque_L/1  "Mot2_Torque_L"
  CANReceive3/2 -> Function-Call Subsystem3/1(CAN_OK)
  CANReceive3/4 -> Function-Call Subsystem3/3(Msg)
  Function-Call Subsystem2/2(Mot1_Sp_L) -> Mot1_Sp_L/1  "Mot1_Sp_L"
  Function-Call Subsystem3/3(Mot2_Torque_H) -> Mot2_Torque_H/1  "Mot2_Torque_H"
  Function-Call Subsystem2/4(Mot1_Torque_L) -> Mot1_Torque_L/1  "Mot1_Torque_L"
  Function-Call Subsystem3/2(Mot2_Sp_L) -> Mot2_Sp_L/1  "Mot2_Sp_L"
  Function-Call Subsystem2/1(Mot1_Sp_H) -> Mot1_Sp_H/1  "Mot1_Sp_H"
  Function-Call Subsystem3/1(Mot2_Sp_H) -> Mot2_Sp_H/1  "Mot2_Sp_H"
  Bus Creator/1 -> Bus Creator2/1
  Bus Creator1/1 -> Bus Creator2/2
  Bus Creator2/1 -> mode_control/1

== system version5/input/MCUtoVCU ==
  CANReceive4 : ec5744lib/RapidECU_U3/04CANCommunication/CANReceive  canmodule=0  canbuffer=2  canmessageid=hex2dec('CFFC7EF')  canmessagetype=Extended(29-bit ID)  datalength=8  sampletime=-1
      settings: SourceProductName=ECUCoder for MPC5744
  CANReceive5 : ec5744lib/RapidECU_U3/04CANCommunication/CANReceive  canmodule=0  canbuffer=0  canmessageid=hex2dec('CB321EF')  canmessagetype=Extended(29-bit ID)  datalength=8  sampletime=-1
      settings: SourceProductName=ECUCoder for MPC5744
  Function-Call Subsystem4 : Subsystem  TreatAsAtomicUnit=on
  Function-Call Subsystem5 : Subsystem  TreatAsAtomicUnit=on
  Terminator4 : Terminator
  Terminator5 : Terminator
  MCU_Temp1 : Outport
  Motor_Temp1 : Outport  Port=2
  MCU_Temp2 : Outport  Port=3
  Motor_Temp2 : Outport  Port=4
  wires:
  CANReceive5/4 -> Function-Call Subsystem5/3(Msg)
  CANReceive4/1 -> Function-Call Subsystem4/Trigger
  CANReceive4/4 -> Function-Call Subsystem4/3(Msg)
  CANReceive5/5 -> Terminator5/1
  CANReceive5/2 -> Function-Call Subsystem5/1(CAN_OK)
  CANReceive4/3 -> Function-Call Subsystem4/2(ID)
  CANReceive5/3 -> Function-Call Subsystem5/2(ID)
  CANReceive5/1 -> Function-Call Subsystem5/Trigger
  CANReceive4/2 -> Function-Call Subsystem4/1(CAN_OK)
  CANReceive4/5 -> Terminator4/1
  Function-Call Subsystem5/1(MCU_Temp2) -> MCU_Temp2/1  "MCU_Temp2"
  Function-Call Subsystem4/1(MCU_Temp1) -> MCU_Temp1/1  "MCU_Temp1"
  Function-Call Subsystem5/2(Motor_Temp2) -> Motor_Temp2/1  "Motor_Temp2"
  Function-Call Subsystem4/2(Motor_Temp1) -> Motor_Temp1/1  "Motor_Temp1"

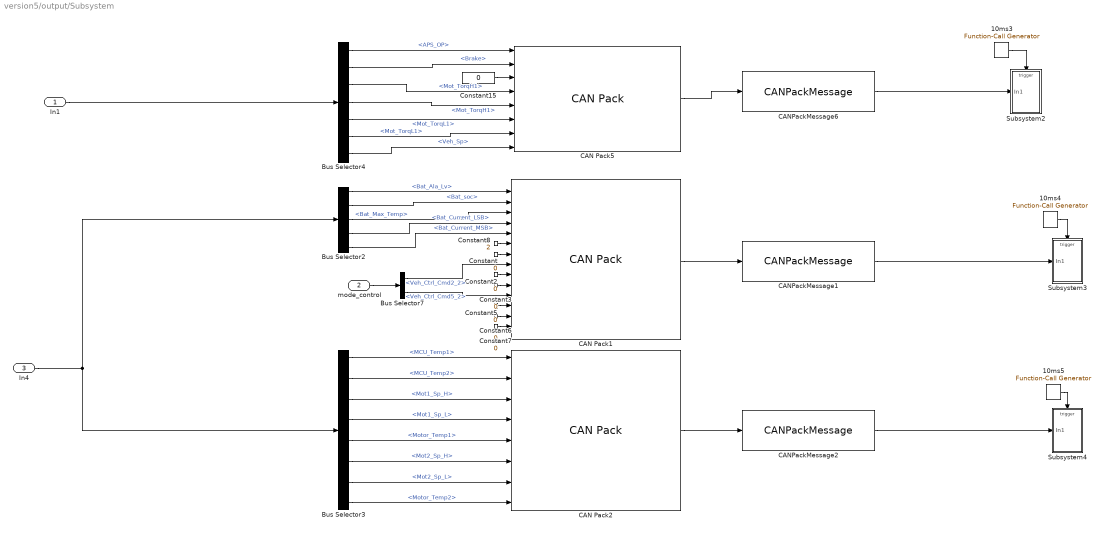
== system version5/output/Subsystem ==
  In1 : Inport
  mode_control : Inport  Port=2
  In4 : Inport  Port=3
  10ms3 : simulink/Ports & Subsystems/Function-Call Generator  sample_time=0.01  numberOfIterations=1
  10ms4 : simulink/Ports & Subsystems/Function-Call Generator  sample_time=0.01  numberOfIterations=1
  10ms5 : simulink/Ports & Subsystems/Function-Call Generator  sample_time=0.01  numberOfIterations=1
  Bus Selector2 : BusSelector  OutputSignals=Bat_Ala_Lv,Bat_soc,Bat_Max_Temp,Bat_Current_LSB,Bat_Current_MSB
  Bus Selector3 : BusSelector  OutputSignals=MCU_Temp1,MCU_Temp2,Mot1_Sp_H,Mot1_Sp_L,Motor_Temp1,Mot2_Sp_H,Mot2_Sp_L,Motor_Temp2
  Bus Selector4 : BusSelector  OutputSignals=APS_OP,Brake,Mot_TorqH1,Mot_TorqH1,Mot_TorqL1,Mot_TorqL1,Veh_Sp
  Bus Selector7 : BusSelector  OutputSignals=signal1.Veh_Ctrl_Cmd2_2,signal1.Veh_Ctrl_Cmd5_2
  CAN Pack1 : canmsglib/CAN Pack  CANdbFile=C:\WH\MC.dbc  MsgList=VCUtoDASH_Bat  MsgName=VCUtoDASH_Bat  MsgIDType=Standard (11-bit identifier)  MsgIdentifier=531  MsgLength=8  SignalInfo=Bat_Ala_Lv$4$4$1$2$1$0$1$0$0$15$#Bat_Soc$16$8$1$2$1$0$1$0$0$255$#Bat_Tp$8$8$1$2$1$0$1$-40$-40$215$#Bat_Voltage_LSB$24$8$1$1$1$0$1.000000e-01$0$0$2.550000e+01$#Bat_Voltage_MSB$32$8$1$1$1$0$1.000000e-01$0$0$2.550000e+01$#Gear_State_Dash$46$2$1$1$1$0$1$0$0$3$#Veh_Ctrl_Cmd1$48$1$1$2$1$0$1$0$0$1$#Veh_Ctrl_Cmd2$49$1$1$2$1$0$1$0$0$1$#Veh_Ctrl_Cmd3$50$1$1$2$1$0$1$0$0$1$#Veh_Ctrl_Cmd4$51$1$1$2$1$0$1$0$0$1$#Veh_Ctrl_Cmd5$52$1$1$2$1$0$1$0$0$1$#Veh_Ctrl_Cmd6$53$1$1$2$1$0$1$0$0$1$#Veh_Ctrl_Cmd7$54$1$1$2$1$0$1$0$0$1$#Veh_Ctrl_Cmd8$55$1$1$2$1$0$1$0$0$1$#  NSignals=14  StartBits=str2num('[int32(4);int32(16);int32(8);int32(24);int32(32);int32(46);int32(48);int32(49);int32(50);int32(51);int32(52);int32(53);int32(54);int32(55)]')  SignalSizes=str2num('[int32(4);int32(8);int32(8);int32(8);int32(8);int32(2);int32(1);int32(1);int32(1);int32(1);int32(1);int32(1);int32(1);int32(1)]')  ByteOrders=str2num('[int32(1);int32(1);int32(1);int32(1);int32(1);int32(1);int32(1);int32(1);int32(1);int32(1);int32(1);int32(1);int32(1);int32(1)]')  DataTypes=str2num('[int32(2);int32(2);int32(2);int32(1);int32(1);int32(1);int32(2);int32(2);int32(2);int32(2);int32(2);int32(2);int32(2);int32(2)]')  MultiplexTypes=str2num('[int32(1);int32(1);int32(1);int32(1);int32(1);int32(1);int32(1);int32(1);int32(1);int32(1);int32(1);int32(1);int32(1);int32(1)]')  MultiplexValues=str2num('[double(0);double(0);double(0);double(0);double(0);double(0);double(0);double(0);double(0);double(0);double(0);double(0);double(0);double(0)]')  Factors=str2num('[double(1);double(1);double(1);double(1.000000e-01);double(1.000000e-01);double(1);double(1);double(1);double(1);double(1);double(1);double(1);double(1);double(1)]')  Offsets=str2num('[double(0);double(0);double(-40);double(0);double(0);double(0);double(0);double(0);double(0);double(0);double(0);double(0);double(0);double(0)]')  Minimums=str2num('[double(0);double(0);double(-40);double(0);double(0);double(0);double(0);double(0);double(0);double(0);double(0);double(0);double(0);double(0)]')  Maximums=str2num('[double(15);double(255);double(215);double(2.550000e+01);double(2.550000e+01);double(3);double(1);double(1);double(1);double(1);double(1);double(1);double(1);double(1)]')  Remote=off  ApplyMinMax=off  BusOutput=off
      settings: SourceProductName=Simulink Real-Time  SourceProductBaseCode=XP  DataFormat=CANdb specified signals
  CAN Pack2 : canmsglib/CAN Pack  CANdbFile=C:\WH\MC.dbc  MsgList=VCUtoDASH_Mot  MsgName=VCUtoDASH_Mot  MsgIDType=Standard (11-bit identifier)  MsgIdentifier=530  MsgLength=8  SignalInfo=Controller1_Temp$24$8$1$2$1$0$1$-50$-50$200$#Controller2_Temp$56$8$1$2$1$0$1$-50$-50$200$#Mot1_Sp_H$0$8$1$2$1$0$5.000000e-01$-10000$-10000$-9.872500e+03$#Mot1_Sp_L$8$8$1$2$1$0$1$-10000$-10000$-9.872500e+03$#Mot1_Tp$16$8$1$2$1$0$1$-50$-50$200$#Mot2_Sp_H$32$8$1$2$1$0$1$-10000$-10000$-9.872500e+03$#Mot2_Sp_L$40$8$1$2$1$0$1$-10000$-10000$-9.872500e+03$#Mot2_Tp$48$8$1$2$1$0$1$-50$-50$200$#  NSignals=8  StartBits=str2num('[int32(24);int32(56);int32(0);int32(8);int32(16);int32(32);int32(40);int32(48)]')  SignalSizes=str2num('[int32(8);int32(8);int32(8);int32(8);int32(8);int32(8);int32(8);int32(8)]')  ByteOrders=str2num('[int32(1);int32(1);int32(1);int32(1);int32(1);int32(1);int32(1);int32(1)]')  DataTypes=str2num('[int32(2);int32(2);int32(2);int32(2);int32(2);int32(2);int32(2);int32(2)]')  MultiplexTypes=str2num('[int32(1);int32(1);int32(1);int32(1);int32(1);int32(1);int32(1);int32(1)]')  MultiplexValues=str2num('[double(0);double(0);double(0);double(0);double(0);double(0);double(0);double(0)]')  Factors=str2num('[double(1);double(1);double(5.000000e-01);double(1);double(1);double(1);double(1);double(1)]')  Offsets=str2num('[double(-50);double(-50);double(-10000);double(-10000);double(-50);double(-10000);double(-10000);double(-50)]')  Minimums=str2num('[double(-50);double(-50);double(-10000);double(-10000);double(-50);double(-10000);double(-10000);double(-50)]')  Maximums=str2num('[double(200);double(200);double(-9.872500e+03);double(-9.872500e+03);double(200);double(-9.872500e+03);double(-9.872500e+03);double(200)]')  Remote=off  ApplyMinMax=off  BusOutput=off
      settings: SourceProductName=Simulink Real-Time  SourceProductBaseCode=XP  DataFormat=CANdb specified signals
  CAN Pack5 : canmsglib/CAN Pack  CANdbFile=C:\WH\MC.dbc  MsgList=VCUtoDASH_Pow  MsgName=VCUtoDASH_Pow  MsgIDType=Standard (11-bit identifier)  MsgIdentifier=529  MsgLength=8  SignalInfo=APS_Op$8$8$1$2$1$0$1$0$0$255$#BPP_Op$16$8$1$2$1$0$1$0$0$255$#Distance$24$8$1$2$1$0$1$0$0$255$#Mot1_Torque_H$32$8$1$2$1$0$1$0$0$255$#Mot1_Torque_L$40$8$1$2$1$0$1$0$0$255$#Mot2_Torque_H$48$8$1$2$1$0$1$0$0$255$#Mot2_Torque_L$56$8$1$2$1$0$1$0$0$255$#Veh_Sp$0$8$1$2$1$0$1$0$0$255$#  NSignals=8  StartBits=str2num('[int32(8);int32(16);int32(24);int32(32);int32(40);int32(48);int32(56);int32(0)]')  SignalSizes=str2num('[int32(8);int32(8);int32(8);int32(8);int32(8);int32(8);int32(8);int32(8)]')  ByteOrders=str2num('[int32(1);int32(1);int32(1);int32(1);int32(1);int32(1);int32(1);int32(1)]')  DataTypes=str2num('[int32(2);int32(2);int32(2);int32(2);int32(2);int32(2);int32(2);int32(2)]')  MultiplexTypes=str2num('[int32(1);int32(1);int32(1);int32(1);int32(1);int32(1);int32(1);int32(1)]')  MultiplexValues=str2num('[double(0);double(0);double(0);double(0);double(0);double(0);double(0);double(0)]')  Factors=str2num('[double(1);double(1);double(1);double(1);double(1);double(1);double(1);double(1)]')  Offsets=str2num('[double(0);double(0);double(0);double(0);double(0);double(0);double(0);double(0)]')  Minimums=str2num('[double(0);double(0);double(0);double(0);double(0);double(0);double(0);double(0)]')  Maximums=str2num('[double(255);double(255);double(255);double(255);double(255);double(255);double(255);double(255)]')  Remote=off  ApplyMinMax=off  BusOutput=off
      settings: SourceProductName=Simulink Real-Time  SourceProductBaseCode=XP  DataFormat=CANdb specified signals
  CANPackMessage1 : ec5744lib/RapidECU_U3/04CANCommunication/CANPackMessage  datalength=8  sampletime=-1
      settings: SourceProductName=ECUCoder for MPC5744
  CANPackMessage2 : ec5744lib/RapidECU_U3/04CANCommunication/CANPackMessage  datalength=8  sampletime=-1
      settings: SourceProductName=ECUCoder for MPC5744
  CANPackMessage6 : ec5744lib/RapidECU_U3/04CANCommunication/CANPackMessage  datalength=8  sampletime=-1
      settings: SourceProductName=ECUCoder for MPC5744
  Constant{,2..3,5..7,15} (7 alike) : Constant  Value=0
  Constant8 : Constant  Value=2
  Subsystem2 : Subsystem
  Subsystem3 : Subsystem
  Subsystem4 : Subsystem
  wires:
  Bus Selector4/4 -> CAN Pack5/5  "<Mot_TorqH1>"
  Bus Selector4/6 -> CAN Pack5/7  "<Mot_TorqL1>"
  Bus Selector4/7 -> CAN Pack5/8  "<Veh_Sp>"
  10ms5/1 -> Subsystem4/Trigger
  In4/1 -> Bus Selector3/1, Bus Selector2/1
  Constant6/1 -> CAN Pack1/13
  Constant15/1 -> CAN Pack5/3
  Bus Selector3/5 -> CAN Pack2/5  "<Motor_Temp1>"
  CAN Pack2/1 -> CANPackMessage2/1
  Constant8/1 -> CAN Pack1/6
  Constant5/1 -> CAN Pack1/12
  Constant2/1 -> CAN Pack1/9
  Bus Selector4/3 -> CAN Pack5/4  "<Mot_TorqH1>"
  Bus Selector4/5 -> CAN Pack5/6  "<Mot_TorqL1>"
  Constant/1 -> CAN Pack1/7
  Constant7/1 -> CAN Pack1/14
  mode_control/1 -> Bus Selector7/1
  Bus Selector3/8 -> CAN Pack2/8  "<Motor_Temp2>"
  Bus Selector3/7 -> CAN Pack2/7  "<Mot2_Sp_L>"
  10ms3/1 -> Subsystem2/Trigger
  Bus Selector2/5 -> CAN Pack1/5  "<Bat_Current_MSB>"
  Bus Selector7/1 -> CAN Pack1/8  "<Veh_Ctrl_Cmd2_2>"
  In1/1 -> Bus Selector4/1
  Bus Selector3/4 -> CAN Pack2/4  "<Mot1_Sp_L>"
  Bus Selector3/3 -> CAN Pack2/3  "<Mot1_Sp_H>"
  CAN Pack1/1 -> CANPackMessage1/1
  Bus Selector2/1 -> CAN Pack1/1  "<Bat_Ala_Lv>"
  Bus Selector2/4 -> CAN Pack1/4  "<Bat_Current_LSB>"
  Bus Selector3/1 -> CAN Pack2/1  "<MCU_Temp1>"
  Bus Selector2/2 -> CAN Pack1/2  "<Bat_soc>"
  10ms4/1 -> Subsystem3/Trigger
  CAN Pack5/1 -> CANPackMessage6/1
  Bus Selector2/3 -> CAN Pack1/3  "<Bat_Max_Temp>"
  Constant3/1 -> CAN Pack1/10
  Bus Selector4/1 -> CAN Pack5/1  "<APS_OP>"
  CANPackMessage6/1 -> Subsystem2/1(In1)
  Bus Selector7/2 -> CAN Pack1/11  "<Veh_Ctrl_Cmd5_2>"
  Bus Selector4/2 -> CAN Pack5/2  "<Brake>"
  Bus Selector3/2 -> CAN Pack2/2  "<MCU_Temp2>"
  Bus Selector3/6 -> CAN Pack2/6  "<Mot2_Sp_H>"
  CANPackMessage2/1 -> Subsystem4/1(In1)
  CANPackMessage1/1 -> Subsystem3/1(In1)
